simulink model "GenerareData"  (R2015b)
settings: Solver=VariableStepAuto  StartTime=0.0  StopTime=30  RelTol=1e-3
libraries: simulink x2
settings Model: Creator=EriveltonDell  LastModifiedBy=EriveltonDell

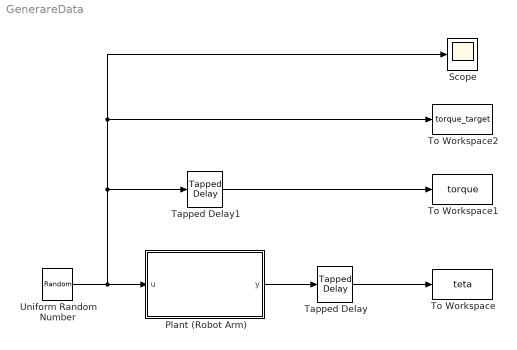
== system GenerareData ==
  Plant (Robot Arm) : Subsystem
      mask Display: plot([-10],[0],[10],[0],[-2 -2 2 2 -2],[5 4 4 5 5],[0 3],[4.5 0.5])
  Scope : Scope
  Tapped Delay : simulink/Discrete/Tapped Delay  vinit=0.0  samptime=-1  NumDelays=4  DelayOrder=Oldest  includeCurrent=off
  Tapped Delay1 : simulink/Discrete/Tapped Delay  vinit=0.0  samptime=-1  NumDelays=4  DelayOrder=Oldest  includeCurrent=off
  To Workspace : ToWorkspace  VariableName=teta  SampleTime=-1
  To Workspace1 : ToWorkspace  VariableName=torque  SampleTime=-1
  To Workspace2 : ToWorkspace  VariableName=torque_target  SampleTime=-1
  Uniform Random Number : UniformRandomNumber  SampleTime=0.1
  wires:
  Plant (Robot Arm)/1(y) -> Tapped Delay/1
  Tapped Delay/1 -> To Workspace/1
  Tapped Delay1/1 -> To Workspace1/1
  Uniform Random Number/1 -> Tapped Delay1/1, To Workspace2/1, Scope/1, Plant (Robot Arm)/1(u)

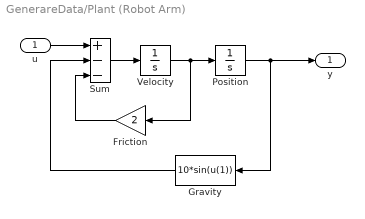
== system GenerareData/Plant (Robot Arm) ==
  u : Inport
  Friction : Gain  Gain=2  SaturateOnIntegerOverflow=on  OutDataTypeStr=Inherit: Same as input  ParamDataTypeStr=Inherit: Same as input
  Gravity : Fcn  Expr=10*sin(u(1))
  Position : Integrator  ZeroCross=off
  Sum : Sum  Inputs=+--  SaturateOnIntegerOverflow=on  InputSameDT=on  OutDataTypeStr=Inherit: Same as first input
  Velocity : Integrator  ZeroCross=off
  y : Outport
  wires:
  Position/1 -> y/1, Gravity/1
  u/1 -> Sum/1
  Sum/1 -> Velocity/1
  Gravity/1 -> Sum/2
  Velocity/1 -> Position/1, Friction/1
  Friction/1 -> Sum/3
